simulink model "array_thd"  (R2014a)
settings: Solver=ode45  StartTime=0.0  StopTime=10.0  RelTol=1e-3
values from neighbouring files (symbols this model uses):
  Ts = Tthd    (= 1.66666666667e-05)    [array_init.m]
libraries: powerlib_meascontrol x3
settings Model: Creator=Taylor  LastModifiedBy=Taylor

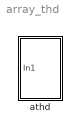
== system array_thd ==
  athd : Subsystem  VariantControl=Variant1

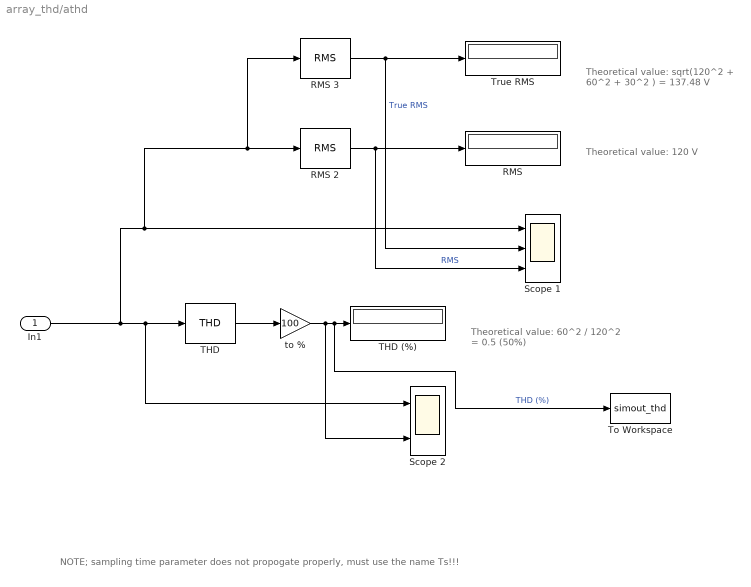
== system array_thd/athd ==
  note: Theoretical value:
      | 120 V
  note: Theoretical value:
      | sqrt(120^2 + 60^2 + 30^2 )
      | = 137.48 V
  note: Theoretical value:
      | 60^2 / 120^2 = 0.5  (50%)
  note: NOTE; sampling time parameter does not propogate properly, must use the name Ts!!!
  In1 : Inport
  RMS : Display
      settings: Format=bank
  RMS 2 : powerlib_meascontrol/Measurements/RMS  TrueRMS=off  Freq=Fgrid  RMSInit=Vgridrms  Ts=Ts
  RMS 3 : powerlib_meascontrol/Measurements/RMS  TrueRMS=on  Freq=Fgrid  RMSInit=Vgridrms  Ts=Ts
  Scope 1 : Scope  NumInputPorts=3
      settings: TimeRange=0.1  YMin=-250~50~50  YMax=250~150~150  SaveName=ScopeData2
  Scope 2 : Scope  NumInputPorts=2
      settings: TimeRange=0.0333333  YMin=-550~0  YMax=500~50
  THD : powerlib_meascontrol/Measurements/THD  Freq=Fgrid  Ts=Ts
  THD (%) : Display
      settings: Format=bank
  To Workspace : ToWorkspace  VariableName=simout_thd  SaveFormat=Timeseries  SampleTime=-1
  True RMS : Display
      settings: Format=bank
  to % : Gain  Gain=100  SampleTime=Ts
  wires:
  RMS 3/1 -> Scope 1/2, True RMS/1  "True RMS"
  RMS 2/1 -> Scope 1/3, RMS/1  "RMS"
  In1/1 -> THD/1, Scope 2/1, Scope 1/1, RMS 3/1, RMS 2/1
  to %/1 -> Scope 2/2, To Workspace/1, THD (%)/1  "THD (%)"
  THD/1 -> to %/1
